simulink model "Ex1"  (R2020a)
settings: Solver=ode23t  StartTime=0.0  StopTime=.1  MaxStep=10^-5  RelTol=1e-3
InitFcn:
  | a=30;
  | m=2;
  | n=1;
libraries: powerlib x6
settings Model: Creator=User  LastModifiedBy=User

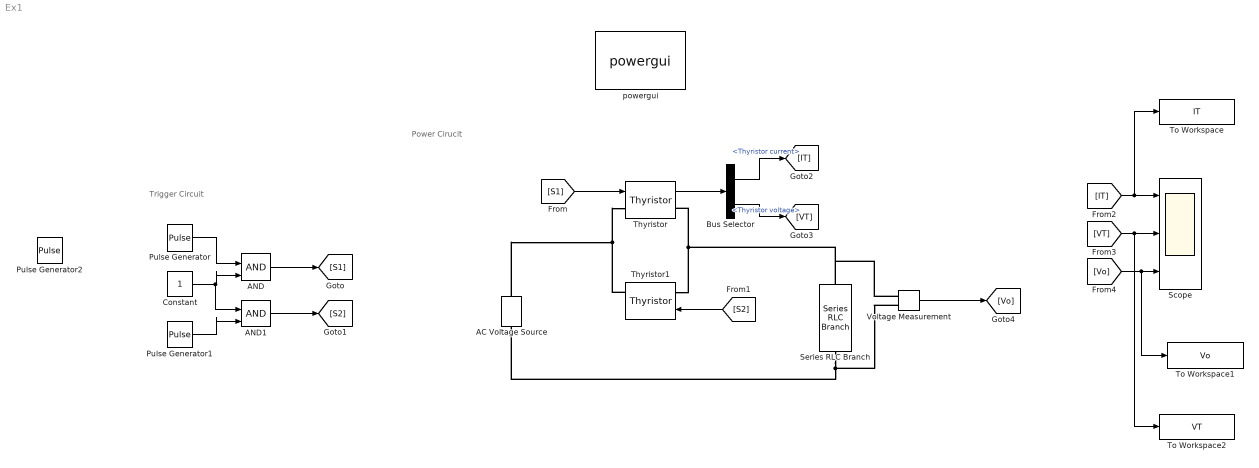
== system Ex1 ==
  note: Trigger Circuit
  note: Power Cirucit
  AC Voltage Source : powerlib/Electrical Sources/AC Voltage Source  Amplitude=100  Phase=0  Frequency=50  SampleTime=0  Measurements=None  BusType=swing  Pref=10e3  Qref=0  Qmin=-inf  Qmax=+inf
  AND : Logic  IconShape=distinctive  AllPortsSameDT=off  OutDataTypeStr=boolean
  AND1 : Logic  IconShape=distinctive  AllPortsSameDT=off  OutDataTypeStr=boolean
  Bus Selector : BusSelector  OutputSignals=Thyristor current,Thyristor voltage
  Constant : Constant
  Pulse Generator : DiscretePulseGenerator  PulseType=Time based  Period=.02  PulseWidth=5  PhaseDelay=(a/360)*.02
  Pulse Generator1 : DiscretePulseGenerator  PulseType=Time based  Period=.02  PulseWidth=5  PhaseDelay=(a/360)*.02+.01
  Pulse Generator2 : DiscretePulseGenerator  PulseType=Time based  Period=.02*(m+n)  PulseWidth=m/(m+n)*100
  Scope : Scope  NumInputPorts=3
  Series RLC Branch : powerlib/Elements/Series RLC Branch  LConnTagsString=__new0  RConnTagsString=__new0  BranchType=R  Resistance=100  Inductance=1e-3  SetiL0=off  InitialCurrent=0  Capacitance=1e-6  Setx0=off  InitialVoltage=0  Measurements=None
  Thyristor : powerlib/Power Electronics/Thyristor  Ron=0.001  Lon=0  Vf=0.8  IC=0  Rs=500  Cs=250e-9  Measurements=on
  Thyristor1 : powerlib/Power Electronics/Thyristor  Ron=0.001  Lon=0  Vf=0.8  IC=0  Rs=500  Cs=250e-9  Measurements=on
  To Workspace : ToWorkspace  VariableName=IT  SampleTime=-1
  To Workspace1 : ToWorkspace  VariableName=Vo  SampleTime=-1
  To Workspace2 : ToWorkspace  VariableName=VT  SampleTime=-1
  Voltage Measurement : powerlib/Measurements/Voltage Measurement  PhasorSimulation=off  OutputType=Complex  PSBequivalent=0
  powergui : powerlib/powergui  Priority=1  SimulationMode=Continuous  SampleTime=50e-6  frequency=60  Iterations=50  frequencyindice=50  Pbase=100e6  ErrMax=1e-4  UnitsV=kV  UnitsW=MW  buscounter=0  FunctionMessages=off  echomessages=off  EnableUseOfTLC=off  CurrentSourceSwitches=off  DisableSnubberDevices=on  DisableRonSwitches=on  DisableVfSwitches=on  DisplayEquations=off  AutomaticDiscreteSolvers=off  SolverType=Tustin/Backward Euler (TBE)  Interpol=off  ExternalGateDelay=off  methode=off  Ts=100  x0status=blocks  SPID=on  SwTol=0  HookPort=off  NonlinearTolerance=1e-4  nMaxIteration=100  ContinueOnMaxIteration=off  RestoreLinks=warning  ResistiveCurrentMeasurement=off  Frange=[0:2:500]  Ylog=off  Xlog=on  ShowGrid=off  save=off  variable=ZData  structure=0  ZoomFFT=off  StartTime=0.0  cycles=1  DisplayStyle=1  fundamental=60  FreqAxis=off  MaxFrequency=1000  frequencyindicesteady=1  RmsSteady=1  display=off
  wires:
  Pulse Generator/1 -> AND/1
  Pulse Generator1/1 -> AND1/2
  AND/1 -> [S1]
  AND1/1 -> [S2]
  [S1] -> Thyristor/1
  [S2] -> Thyristor1/1
  Thyristor/1 -> Bus Selector/1
  Bus Selector/1 -> [IT]  "<Thyristor current>"
  Bus Selector/2 -> [VT]  "<Thyristor voltage>"
  Voltage Measurement/1 -> [Vo]
  [IT] -> To Workspace/1, Scope/1
  [VT] -> To Workspace2/1, Scope/2
  [Vo] -> To Workspace1/1, Scope/3
  Constant/1 -> AND1/1, AND/2
  connections:
  Thyristor1/LConn1 -- Voltage Measurement/LConn1 -- Series RLC Branch/LConn1 -- Thyristor/RConn1
  Thyristor1/RConn1 -- AC Voltage Source/RConn1 -- Thyristor/LConn1
  Series RLC Branch/RConn1 -- Voltage Measurement/LConn2 -- AC Voltage Source/LConn1
